simulink model "CAE_11"  (R2018b)
settings: Solver=ode4  StartTime=0.0  StopTime=1.6  FixedStep=fixed_step_size  RelTol=1e-3  EnableMultiTasking=on
values from neighbouring files (symbols this model uses):
  amax = 600    [CAE_11_v_1.m]    (also in CAE_14_v1.M; CAE_14d.m)
  coeff = 1    [CAE_11_v_1.m]    (also in CAE_14d.m)
  dm = 0.1    [CAE_10_v1.m]    (also in CAE_11_v_1.m; CAE_14_v1.M; CAE_14d.m; CAE_8_v1.m)
  t1 = .2    (= 0.2)    [CAE_11_v_1.m]    (also in CAE_14_v1.M; CAE_14d.m)
  teqt = 1.5*Tt+Tew+Tfw    (= 0.0312)    [CAE_10_v1.m]    (also in CAE_11_v_1.m; CAE_14_v1.M = 0.031192; CAE_14d.m = 0.031192; CAE_8_v1.m)
  teta0 = 0    [BLAC1_v1.m]    (also in BLAC1_v2.m; CAE_11_v_1.m; CAE_14_v1.M; CAE_14d.m)
  tl = 0.4    [CAE_11_v_1.m]    (also in CAE_14_v1.M; CAE_14d.m)
  tr = .0001    (= 0.0001)    [CAE_11_v_1.m]    (also in CAE_14_v1.M = 0; CAE_14d.m)
  wom = 8*2*pi    (= 50.2654824574)    [CAE_10_v1.m]    (also in CAE_11_v_1.m; CAE_14_v1.M; CAE_14d.m; CAE_8_v1.m)
libraries: simulink x1
settings Model: Creator=Francesco  LastModifiedBy=anton
settings DataIOCC: LimitDataPoints=on  SaveFormat=Array  SignalLoggingSaveFormat=ModelDataLogs
settings OptimizationCC: ExpressionDepthLimit=2147483647  InitFltsAndDblsToZero=on  LifeSpan=inf
settings DebuggingCC: SaveWithParameterizedLinksMsg=none  UnderspecifiedInitializationDetection=Classic  MergeDetectMultiDrivingBlocksExec=none  SignalResolutionControl=TryResolveAllWithWarning  SolverPrmCheckMsg=warning  MultiTaskDSMMsg=warning  MultiTaskCondExecSysMsg=none  FcnCallInpInsideContextMsg=warning  StateNameClashWarn=warning  SFUnexpectedBacktrackingDiag=warning  SFNoUnconditionalDefaultTransitionDiag=warning  SFExecutionAtInitializationDiag=none
settings HardwareCC: ProdBitPerPointer=32  ProdBitPerSizeT=32  ProdBitPerPtrDiffT=32  ProdLargestAtomicFloat=None  ProdIntDivRoundTo=Undefined  ProdEndianess=Unspecified  ProdWordSize=32  ProdHWDeviceType=32-bit Generic
settings ModelReferenceCC: PropagateSignalLabelsOutOfModel=off
settings SFSimCC: SimUseLocalCustomCode=off
settings RTWCC: RTWUseLocalCustomCode=off
settings CodeAppCC: StateflowObjectComments=on
settings GRTTargetCC: TargetFcnLib=ansi_tfl_tmw.mat  TargetLangStandard=C89/C90 (ANSI)  CombineOutputUpdateFcns=off  GRTInterface=on
settings ConfigComp: CovMetricSettings=dw  CovHtmlReporting=on  CovSaveCumulativeToWorkspaceVar=on  CovSaveSingleToWorkspaceVar=on  CovExternalEMLEnable=off

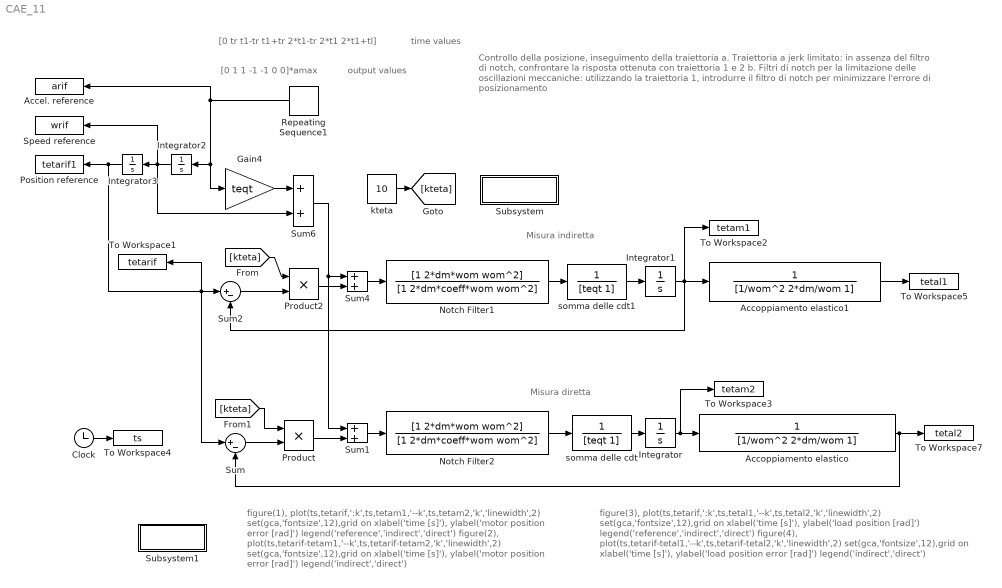
== system CAE_11 ==
  note: Misura indiretta
  note: Misura diretta
  note: Controllo della posizione, inseguimento della traiettoria
      |
      | a. Traiettoria a jerk limitato:
      | in assenza del filtro di notch, confrontare la risposta ottenuta con traiettoria 1 e 2
      |
      | b. Filtri di notch per la limitazione delle oscillazioni meccaniche:
      | utilizzando la traiettoria 1, introdurre il filtro di notch per minimizzare l'errore di posizionamento
  note: figure(3),
      | plot(ts,tetarif,':k',ts,tetal1,'--k',ts,tetal2,'k','linewidth',2)
      | set(gca,'fontsize',12),grid on
      | xlabel('time [s]'), ylabel('load position [rad]')
      | legend('reference','indirect','direct')
      |
      | figure(4),
      | plot(ts,tetarif-tetal1,'--k',ts,tetarif-tetal2,'k','linewidth',2)
      | set(gca,'fontsize',12),grid on
      | xlabel('time [s]'), ylabel('load position error [rad]')
      | legend('indirect','direct')
  note: figure(1),
      | plot(ts,tetarif,':k',ts,tetam1,'--k',ts,tetam2,'k','linewidth',2)
      | set(gca,'fontsize',12),grid on
      | xlabel('time [s]'), ylabel('motor position error [rad]')
      | legend('reference','indirect','direct')
      |
      | figure(2),
      | plot(ts,tetarif-tetam1,'--k',ts,tetarif-tetam2,'k','linewidth',2)
      | set(gca,'fontsize',12),grid on
      | xlabel('time [s]'), ylabel('motor position error [rad]')
      | legend('indirect','direct')
  note: output values
  note: [0 1 1 -1 -1 0 0]*amax
  note: [0 tr t1-tr t1+tr 2*t1-tr 2*t1 2*t1+tl]
  note: time values
  Accel. reference : ToWorkspace  VariableName=arif
      settings: MaxDataPoints=1e6
      settings: OpenFcn=|
      | figure(5);
      | plot(ts,arif,'k','linewidth',2)
      | xlabel('time [s]');
      | ylabel('acceleration [rad/s^2]');
      | title('acceleration trajectory')
  Accoppiamento elastico : TransferFcn  Denominator=[1/wom^2 2*dm/wom 1]
  Accoppiamento elastico1 : TransferFcn  Denominator=[1/wom^2 2*dm/wom 1]
  Clock : Clock
  Gain4 : Gain  Gain=teqt  SaturateOnIntegerOverflow=on  OutDataTypeStr=Inherit: Same as input  ParamDataTypeStr=Inherit: Same as input
  Integrator : Integrator
  Integrator1 : Integrator
  Integrator2 : Integrator
  Integrator3 : Integrator  InitialCondition=teta0
  Notch Filter1 : TransferFcn  Numerator=[1 2*dm*wom wom^2]  Denominator=[1 2*dm*coeff*wom wom^2]
  Notch Filter2 : TransferFcn  Numerator=[1 2*dm*wom wom^2]  Denominator=[1 2*dm*coeff*wom wom^2]
  Position reference : ToWorkspace  VariableName=tetarif1
      settings: MaxDataPoints=1e6
  Product : Product  RndMeth=Zero
  Product2 : Product  RndMeth=Zero
  Repeating Sequence1 : simulink/Sources/Repeating Sequence  rep_seq_t=[0 tr t1-tr t1+tr 2*t1-tr 2*t1 2*t1+tl]  rep_seq_y=[0 1 1 -1 -1 0 0]*amax
  Speed reference : ToWorkspace  VariableName=wrif
      settings: MaxDataPoints=1e6
  Subsystem : Subsystem
      settings: OpenFcn=CAE_11d_2013
      mask Display: disp('LOAD DATA')
  Subsystem1 : Subsystem
      settings: OpenFcn=|
      | figure(1),
      | plot(ts,tetarif,':k',ts,tetam1,'--k',ts,tetam2,'k','linewidth',2)
      | set(gca,'fontsize',12),grid on
      | xlabel('time [s]')
      | ylabel('motor position [rad]')
      | legend('reference','indirect','direct')
      | 
      | figure(2),
      | plot(ts,tetarif-tetam1,'--k',ts,tetarif-tetam2,'k','linewidth',2)
      | set(gca,'fontsize',12),grid on
      | xlabel('time [s]')
      | ylabel('motor position error [rad]')
      | legend('indirect','direct')
      | figure(3),
      | plot(ts,tetarif,':k',ts,tetal1,'--k',ts,tetal2,'k','linewidth',2)
      | set(gca,'fontsize',12),grid on
      | xlabel('time [s]')
      | ylabel('load position [rad]')
      | legend('reference','indirect','direct')
      | 
      | figure(4),
      | plot(ts,tetarif-tetal1,'--k',ts,tetarif-tetal2,'k','linewidth',2)
      | set(gca,'fontsize',12),grid on
      | xlabel('time [s]')
      | ylabel('load position error [rad]')
      | legend('indirect','direct')
      mask Display: disp('grafici')
  Sum : Sum  Inputs=|+-
  Sum1 : Sum  SaturateOnIntegerOverflow=on  InputSameDT=on  OutDataTypeStr=Inherit: Same as first input
  Sum2 : Sum  Inputs=|+-
  Sum4 : Sum  SaturateOnIntegerOverflow=on  InputSameDT=on  OutDataTypeStr=Inherit: Same as first input
  Sum6 : Sum  SaturateOnIntegerOverflow=on  InputSameDT=on  OutDataTypeStr=Inherit: Same as first input
  To Workspace1 : ToWorkspace  VariableName=tetarif
  To Workspace2 : ToWorkspace  VariableName=tetam1
  To Workspace3 : ToWorkspace  VariableName=tetam2
  To Workspace4 : ToWorkspace  VariableName=ts
  To Workspace5 : ToWorkspace  VariableName=tetal1
  To Workspace7 : ToWorkspace  VariableName=tetal2
  kteta : Constant  Value=10
  somma delle cdt : TransferFcn  Denominator=[teqt 1]
  somma delle cdt1 : TransferFcn  Denominator=[teqt 1]
  wires:
  Sum/1 -> Product/2
  somma delle cdt/1 -> Integrator/1
  Integrator/1 -> Accoppiamento elastico/1, To Workspace3/1
  Accoppiamento elastico/1 -> Sum/2, To Workspace7/1
  Sum2/1 -> Product2/2
  somma delle cdt1/1 -> Integrator1/1
  Integrator1/1 -> Accoppiamento elastico1/1, Sum2/2, To Workspace2/1
  Accoppiamento elastico1/1 -> To Workspace5/1
  kteta/1 -> [kteta]
  [kteta] -> Product2/1
  [kteta] -> Product/1
  Clock/1 -> To Workspace4/1
  Integrator2/1 -> Integrator3/1, Speed reference/1, Sum6/2
  Integrator3/1 -> Position reference/1, Sum/1, Sum2/1, To Workspace1/1
  Sum6/1 -> Sum4/1, Sum1/1
  Product2/1 -> Sum4/2
  Repeating Sequence1/1 -> Integrator2/1, Gain4/1, Accel. reference/1
  Product/1 -> Sum1/2
  Gain4/1 -> Sum6/1
  Sum4/1 -> Notch Filter1/1
  Notch Filter1/1 -> somma delle cdt1/1
  Sum1/1 -> Notch Filter2/1
  Notch Filter2/1 -> somma delle cdt/1

== system CAE_11/Subsystem ==

== system CAE_11/Subsystem1 ==
